simulink model "h3p1_sim"  (R2022b)
settings: Solver=VariableStepAuto  StartTime=0.0  StopTime=Tf  RelTol=1e-3
undefined symbols (not defined in the file): J, Jw, kd_pitch, kd_roll, kd_yaw, kp_pitch, kp_roll, kp_yaw, mu, q_inertial2body_0, q_inertial2body_f, r_inertial_0, v_inertial_0, w_b_0, w_b_nom, X_rw_in_body
libraries: matrix_library x1
settings Model: Creator=corey  LastModifiedBy=corey
settings DebuggingCC: UnconnectedInputMsg=warning  UnconnectedOutputMsg=warning  UnconnectedLineMsg=warning
settings ModelReferenceCC: EnableRefExpFcnMdlSchedulingChecks=on
settings RTWCC: DLArmComputeVersion=19.05

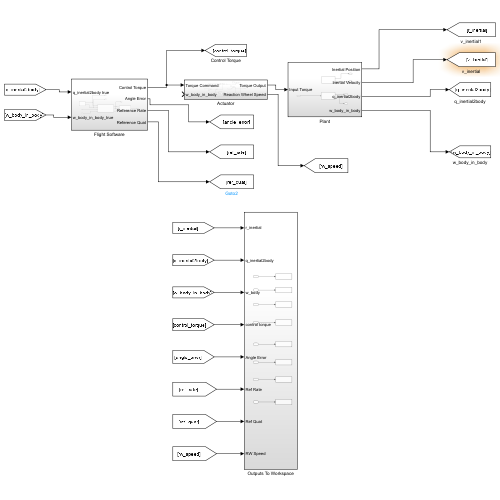
[thumbnail: Simulink's stored preview of the top-level diagram]
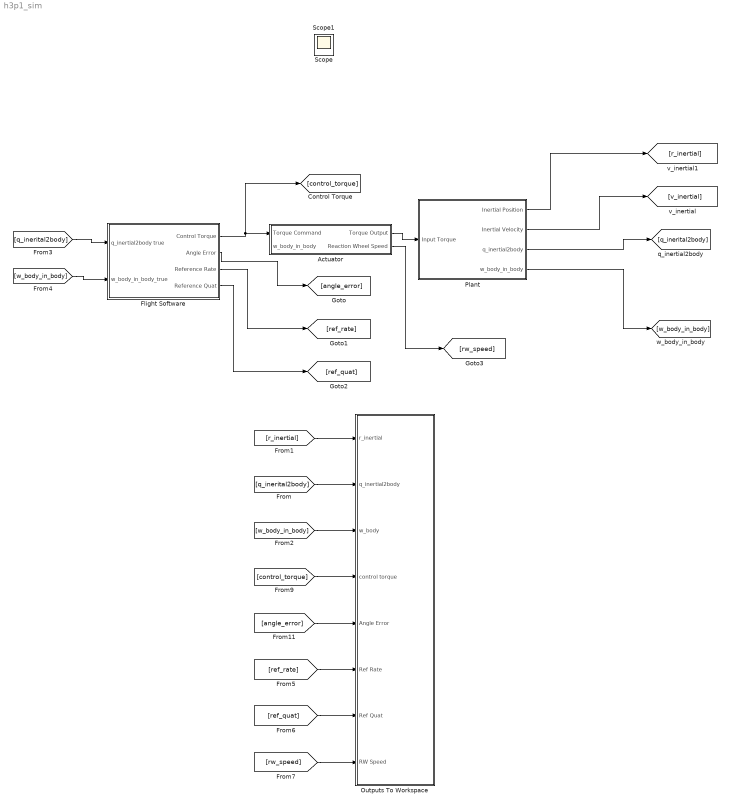
== system h3p1_sim ==
  Actuator : Subsystem
  Flight Software : Subsystem
  Outputs To Workspace : Subsystem
  Plant : Subsystem
  Scope : Scope
  Scope1 : Scope
  wires:
  Plant/4(w_body_in_body) -> [w_body_in_body]
  Plant/3(q_inertial2body) -> [q_inerital2body]
  Plant/2(Inertial Velocity) -> [v_inertial]
  Plant/1(Inertial Position) -> [r_inertial]
  [q_inerital2body] -> Outputs To Workspace/2(q_inertial2body)
  [w_body_in_body] -> Outputs To Workspace/3(w_body)
  [r_inertial] -> Outputs To Workspace/1(r_inertial)
  [control_torque] -> Outputs To Workspace/4(control torque)
  Flight Software/1(Control Torque) -> Actuator/1(Torque Command), [control_torque]
  [angle_error] -> Outputs To Workspace/5(Angle Error)
  Actuator/1(Torque Output) -> Plant/1(Input Torque)
  Flight Software/2(Angle Error) -> [angle_error]
  [q_inerital2body] -> Flight Software/1(q_inertial2body true)
  [w_body_in_body] -> Flight Software/2(w_body_in_body_true)
  Flight Software/3(Reference Rate) -> [ref_rate]
  Flight Software/4(Reference Quat) -> [ref_quat]
  [ref_rate] -> Outputs To Workspace/6(Ref Rate)
  [ref_quat] -> Outputs To Workspace/7(Ref Quat)
  Actuator/2(Reaction Wheel Speed) -> [rw_speed]
  [rw_speed] -> Outputs To Workspace/8(RW Speed)

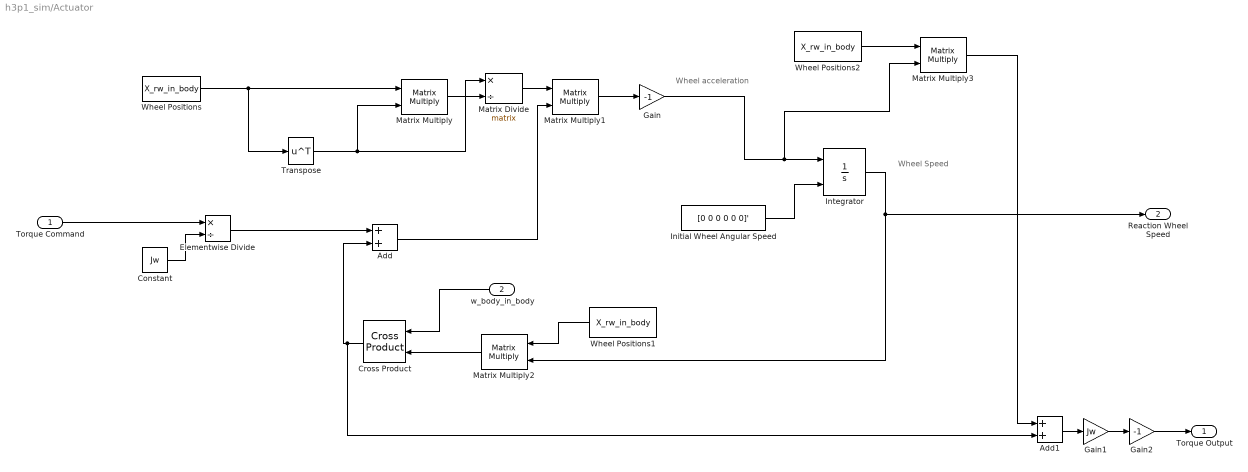
== system h3p1_sim/Actuator ==
  note: Wheel Speed
  note: Wheel acceleration
  Torque Command : Inport
  w_body_in_body : Inport  Port=2
  Add : Sum
  Add1 : Sum
  Constant : Constant  Value=Jw
  Cross Product : matrix_library/Cross Product
  Elementwise Divide : Product  Inputs=*/
  Gain : Gain  Gain=-1
  Gain1 : Gain  Gain=Jw
  Gain2 : Gain  Gain=-1
  Initial Wheel Angular Speed : Constant  Value=[0 0 0 0 0 0]'
  Integrator : Integrator  InitialConditionSource=external
  Matrix Divide : Product  Inputs=*/  Multiplication=Matrix(*)
  Matrix Multiply{,1..3} (4 alike) : Product  Multiplication=Matrix(*)
  Transpose : Math  Operator=transpose
  Wheel Positions : Constant  Value=X_rw_in_body
  Wheel Positions1 : Constant  Value=X_rw_in_body
  Wheel Positions2 : Constant  Value=X_rw_in_body
  Torque Output : Outport
  Reaction Wheel Speed : Outport  Port=2
  wires:
  Initial Wheel Angular Speed/1 -> Integrator/2
  Wheel Positions/1 -> Matrix Multiply/1, Transpose/1
  Transpose/1 -> Matrix Divide/1, Matrix Multiply/2
  Matrix Multiply/1 -> Matrix Divide/2
  Matrix Divide/1 -> Matrix Multiply1/1
  Torque Command/1 -> Elementwise Divide/1
  Constant/1 -> Elementwise Divide/2
  Elementwise Divide/1 -> Add/1
  Integrator/1 -> Reaction Wheel Speed/1, Matrix Multiply2/2
  Wheel Positions1/1 -> Matrix Multiply2/1
  w_body_in_body/1 -> Cross Product/1
  Matrix Multiply2/1 -> Cross Product/2
  Add/1 -> Matrix Multiply1/2
  Matrix Multiply1/1 -> Gain/1
  Gain/1 -> Matrix Multiply3/2, Integrator/1
  Cross Product/1 -> Add1/2, Add/2
  Add1/1 -> Gain1/1
  Wheel Positions2/1 -> Matrix Multiply3/1
  Matrix Multiply3/1 -> Add1/1
  Gain1/1 -> Gain2/1
  Gain2/1 -> Torque Output/1

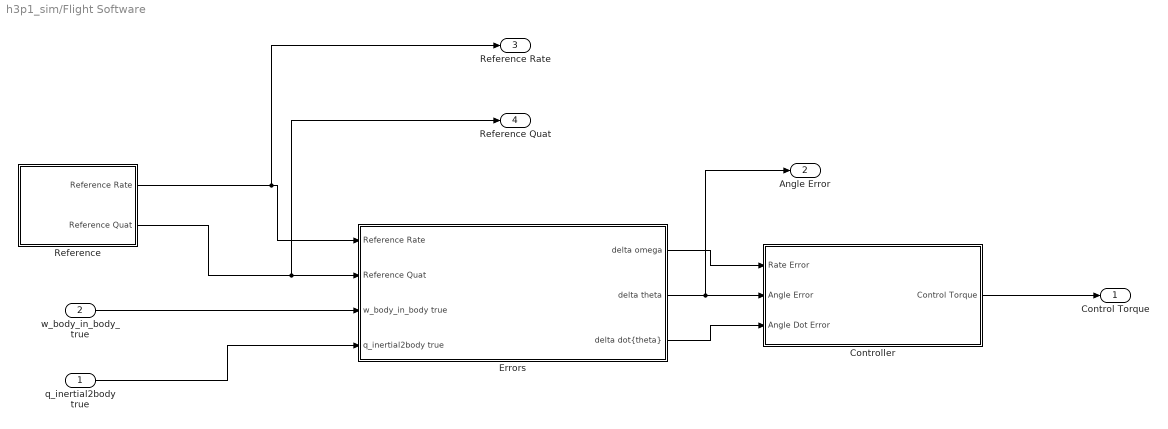
== system h3p1_sim/Flight Software ==
  q_inertial2body true : Inport
  w_body_in_body_true : Inport  Port=2
  Controller : Subsystem
  Errors : Subsystem
  Reference : Subsystem
  Control Torque : Outport
  Angle Error : Outport  Port=2
  Reference Rate : Outport  Port=3
  Reference Quat : Outport  Port=4
  wires:
  Controller/1(Control Torque) -> Control Torque/1
  Errors/1(delta omega) -> Controller/1(Rate Error)
  Errors/2(delta theta) -> Angle Error/1, Controller/2(Angle Error)
  Errors/3("delta dot{theta}") -> Controller/3(Angle Dot Error)
  q_inertial2body true/1 -> Errors/4(q_inertial2body true)
  w_body_in_body_true/1 -> Errors/3(w_body_in_body true)
  Reference/1(Reference Rate) -> Reference Rate/1, Errors/1(Reference Rate)
  Reference/2(Reference Quat) -> Reference Quat/1, Errors/2(Reference Quat)

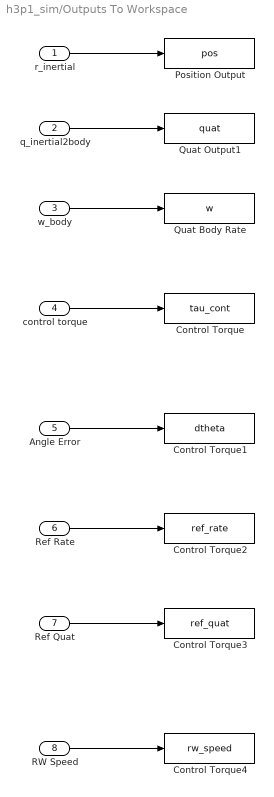
== system h3p1_sim/Outputs To Workspace ==
  r_inertial : Inport
  q_inertial2body : Inport  Port=2
  w_body : Inport  Port=3
  control torque : Inport  Port=4
  Angle Error : Inport  Port=5
  Ref Rate : Inport  Port=6
  Ref Quat : Inport  Port=7
  RW Speed : Inport  Port=8
  Control Torque : ToWorkspace  VariableName=tau_cont  SampleTime=-1
  Control Torque1 : ToWorkspace  VariableName=dtheta  SampleTime=-1
  Control Torque2 : ToWorkspace  VariableName=ref_rate  SampleTime=-1
  Control Torque3 : ToWorkspace  VariableName=ref_quat  SampleTime=-1
  Control Torque4 : ToWorkspace  VariableName=rw_speed  SampleTime=-1
  Position Output : ToWorkspace  VariableName=pos  SampleTime=-1
  Quat Body Rate : ToWorkspace  VariableName=w  SampleTime=-1
  Quat Output1 : ToWorkspace  VariableName=quat  SampleTime=-1
  wires:
  r_inertial/1 -> Position Output/1
  w_body/1 -> Quat Body Rate/1
  q_inertial2body/1 -> Quat Output1/1
  control torque/1 -> Control Torque/1
  Angle Error/1 -> Control Torque1/1
  Ref Rate/1 -> Control Torque2/1
  Ref Quat/1 -> Control Torque3/1
  RW Speed/1 -> Control Torque4/1

== system h3p1_sim/Plant ==
  Input Torque : Inport
  Attitude Dynamics : Subsystem
  Position Dynamics : Subsystem
  Inertial Position : Outport
  Inertial Velocity : Outport  Port=2
  q_inertial2body : Outport  Port=3
  w_body_in_body : Outport  Port=4
  wires:
  Input Torque/1 -> Attitude Dynamics/1(Input Torque)
  Position Dynamics/1(Inertial Position) -> Inertial Position/1
  Position Dynamics/2(Inertial Velocity) -> Inertial Velocity/1
  Attitude Dynamics/1(q_inertial2body) -> q_inertial2body/1
  Attitude Dynamics/2(w_body_in_body) -> w_body_in_body/1

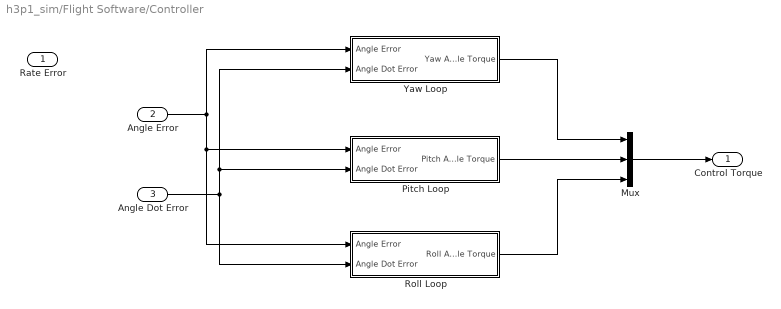
== system h3p1_sim/Flight Software/Controller ==
  Rate Error : Inport
  Angle Error : Inport  Port=2
  Angle Dot Error : Inport  Port=3
  Mux : Mux  Inputs=3
  Pitch Loop : Subsystem
  Roll Loop : Subsystem
  Yaw Loop : Subsystem
  Control Torque : Outport
  wires:
  Angle Error/1 -> Pitch Loop/1(Angle Error), Roll Loop/1(Angle Error), Yaw Loop/1(Angle Error)
  Angle Dot Error/1 -> Pitch Loop/2(Angle Dot Error), Yaw Loop/2(Angle Dot Error), Roll Loop/2(Angle Dot Error)
  Mux/1 -> Control Torque/1
  Yaw Loop/1(Yaw Angle Torque) -> Mux/1
  Pitch Loop/1(Pitch Angle Torque) -> Mux/2
  Roll Loop/1(Roll Angle Torque) -> Mux/3

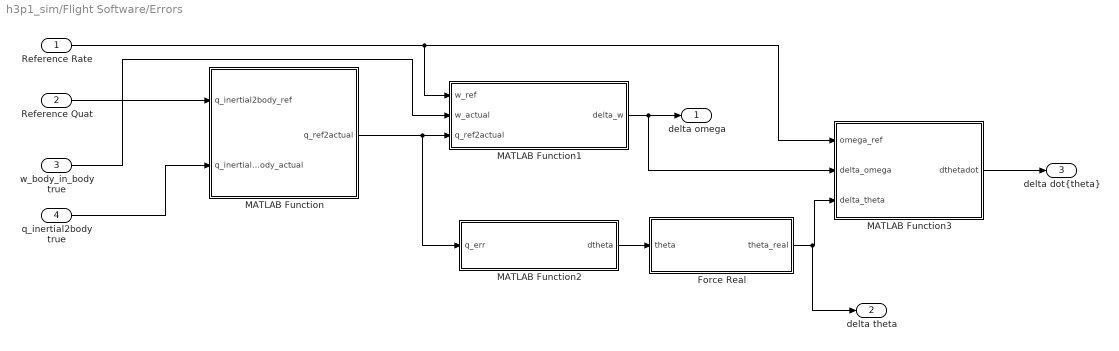
== system h3p1_sim/Flight Software/Errors ==
  Reference Rate : Inport
  Reference Quat : Inport  Port=2
  w_body_in_body true : Inport  Port=3
  q_inertial2body true : Inport  Port=4
  Force Real : MATLAB Function  TreatAsAtomicUnit=on
  MATLAB Function : MATLAB Function  TreatAsAtomicUnit=on
  MATLAB Function1 : MATLAB Function  TreatAsAtomicUnit=on
  MATLAB Function2 : MATLAB Function  TreatAsAtomicUnit=on
  MATLAB Function3 : MATLAB Function  TreatAsAtomicUnit=on
  delta omega : Outport
  delta theta : Outport  Port=2
  "delta dot{theta}" : Outport  Port=3
  wires:
  Reference Quat/1 -> MATLAB Function/1(q_inertial2body_ref)
  q_inertial2body true/1 -> MATLAB Function/2(q_inertial2body_actual)
  MATLAB Function/1(q_ref2actual) -> MATLAB Function2/1(q_err), MATLAB Function1/3(q_ref2actual)
  Reference Rate/1 -> MATLAB Function3/1(omega_ref), MATLAB Function1/1(w_ref)
  w_body_in_body true/1 -> MATLAB Function1/2(w_actual)
  MATLAB Function1/1(delta_w) -> MATLAB Function3/2(delta_omega), delta omega/1
  MATLAB Function3/1(dthetadot) -> "delta dot{theta}"/1
  MATLAB Function2/1(dtheta) -> Force Real/1(theta)
  Force Real/1(theta_real) -> delta theta/1, MATLAB Function3/3(delta_theta)

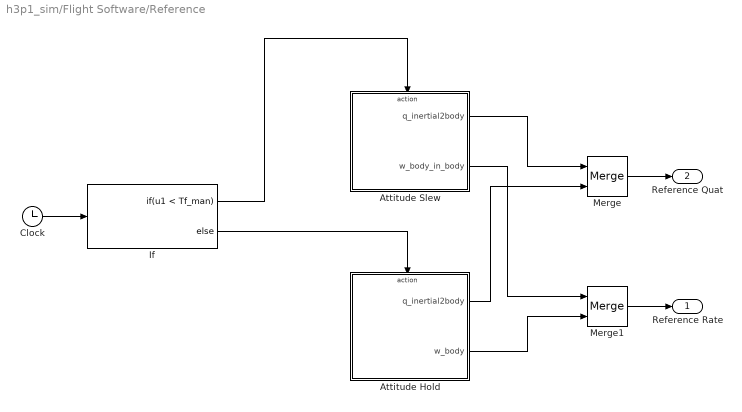
== system h3p1_sim/Flight Software/Reference ==
  Attitude Hold : Subsystem  TreatAsAtomicUnit=on
  Attitude Slew : Subsystem  TreatAsAtomicUnit=on
  Clock : Clock
  If : If  IfExpression=u1 < Tf_man
  Merge : Merge
  Merge1 : Merge
  Reference Rate : Outport
  Reference Quat : Outport  Port=2
  wires:
  Clock/1 -> If/1
  If/1 -> Attitude Slew/Action
  If/2 -> Attitude Hold/Action
  Attitude Slew/1(q_inertial2body) -> Merge/1
  Attitude Hold/1(q_inertial2body) -> Merge/2
  Merge/1 -> Reference Quat/1
  Merge1/1 -> Reference Rate/1
  Attitude Slew/2(w_body_in_body) -> Merge1/1
  Attitude Hold/2(w_body) -> Merge1/2

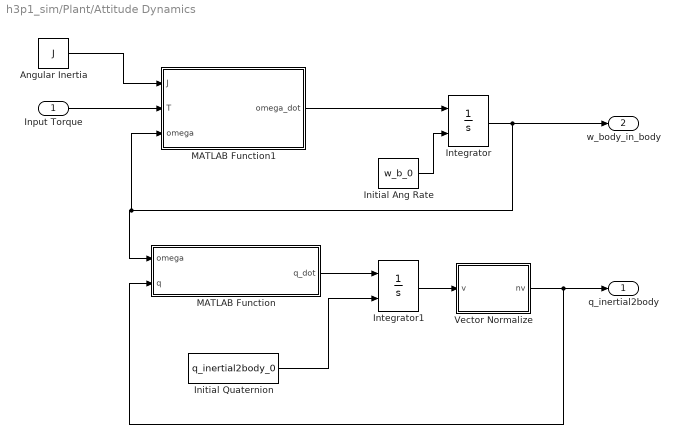
== system h3p1_sim/Plant/Attitude Dynamics ==
  Input Torque : Inport
  Angular Inertia : Constant  Value=J
  Initial Ang Rate : Constant  Value=w_b_0
  Initial Quaternion : Constant  Value=q_inertial2body_0
  Integrator : Integrator  InitialConditionSource=external
  Integrator1 : Integrator  InitialConditionSource=external
  MATLAB Function : MATLAB Function  TreatAsAtomicUnit=on
  MATLAB Function1 : MATLAB Function  TreatAsAtomicUnit=on
  Vector Normalize : MATLAB Function  TreatAsAtomicUnit=on
  q_inertial2body : Outport
  w_body_in_body : Outport  Port=2
  wires:
  Integrator/1 -> MATLAB Function1/3(omega), MATLAB Function/1(omega), w_body_in_body/1
  MATLAB Function1/1(omega_dot) -> Integrator/1
  Initial Ang Rate/1 -> Integrator/2
  MATLAB Function/1(q_dot) -> Integrator1/1
  Initial Quaternion/1 -> Integrator1/2
  Integrator1/1 -> Vector Normalize/1(v)
  Vector Normalize/1(nv) -> MATLAB Function/2(q), q_inertial2body/1
  Input Torque/1 -> MATLAB Function1/2(T)
  Angular Inertia/1 -> MATLAB Function1/1(J)

== system h3p1_sim/Plant/Position Dynamics ==
  Gravity Constant : Constant  Value=mu
  Initial Position : Constant  Value=r_inertial_0
  Initial Velocity : Constant  Value=v_inertial_0
  Integrator : Integrator  InitialConditionSource=external  InitialCondition=[6871, 0, 0]'
  Integrator1 : Integrator  InitialConditionSource=external  InitialCondition=[0, 7.6166, 0]'
  Vector Norm : MATLAB Function  TreatAsAtomicUnit=on
  Inertial Position : Outport
  Inertial Velocity : Outport  Port=2
  wires:
  Integrator/1 -> Vector Norm/1(r), Inertial Position/1  "Position"
  Integrator1/1 -> Inertial Velocity/1, Integrator/1  "Velocity"
  Vector Norm/1(a) -> Integrator1/1  "Accel"
  Gravity Constant/1 -> Vector Norm/2(mu)
  Initial Velocity/1 -> Integrator1/2
  Initial Position/1 -> Integrator/2

== system h3p1_sim/Flight Software/Controller/Pitch Loop ==
  Angle Error : Inport
  Angle Dot Error : Inport  Port=2
  PD Controller : Subsystem
  Pitch Angle Torque : Outport
  wires:
  Angle Error/1 -> PD Controller/1(Angle Error)
  Angle Dot Error/1 -> PD Controller/2(Angle Error Dot)
  PD Controller/1(Pitch Angle Torque) -> Pitch Angle Torque/1

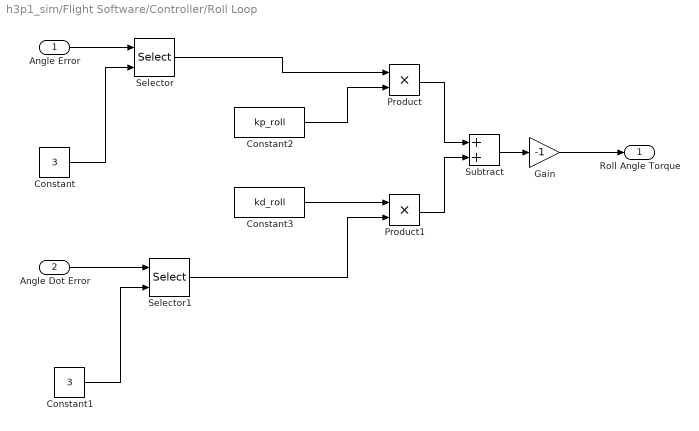
== system h3p1_sim/Flight Software/Controller/Roll Loop ==
  Angle Error : Inport
  Angle Dot Error : Inport  Port=2
  Constant : Constant  Value=3
  Constant1 : Constant  Value=3
  Constant2 : Constant  Value=kp_roll
  Constant3 : Constant  Value=kd_roll
  Gain : Gain  Gain=-1
  Product : Product
  Product1 : Product
  Selector : Selector  InputPortWidth=3  IndexOptions=Index vector (port)  Indices=[1 3]  OutputSizes=1
  Selector1 : Selector  InputPortWidth=3  IndexOptions=Index vector (port)  Indices=[1 3]  OutputSizes=1
  Subtract : Sum
  Roll Angle Torque : Outport
  wires:
  Angle Error/1 -> Selector/1
  Constant/1 -> Selector/2
  Constant1/1 -> Selector1/2
  Angle Dot Error/1 -> Selector1/1
  Selector/1 -> Product/1
  Constant2/1 -> Product/2
  Constant3/1 -> Product1/1
  Selector1/1 -> Product1/2
  Product/1 -> Subtract/1
  Product1/1 -> Subtract/2
  Subtract/1 -> Gain/1
  Gain/1 -> Roll Angle Torque/1

== system h3p1_sim/Flight Software/Controller/Yaw Loop ==
  Angle Error : Inport
  Angle Dot Error : Inport  Port=2
  PD Controller : Subsystem
  Yaw Angle Torque : Outport
  wires:
  Angle Error/1 -> PD Controller/1(Angle Error)
  Angle Dot Error/1 -> PD Controller/2(Angle Error Dot)
  PD Controller/1(Yaw Angle Torque) -> Yaw Angle Torque/1

== system h3p1_sim/Flight Software/Reference/Attitude Hold ==
  Action Port : ActionPort  ActionPortLabel=else
  Constant : Constant  Value=q_inertial2body_f
  Constant1 : Constant  Value=[0 0 0]'
  q_inertial2body : Outport
  w_body : Outport  Port=2
  wires:
  Constant/1 -> q_inertial2body/1
  Constant1/1 -> w_body/1

== system h3p1_sim/Flight Software/Reference/Attitude Slew ==
  Action Port : ActionPort  ActionPortLabel=if(u1 < Tf_man)
  Constant : Constant  Value=[0 0 0]'
  Reference Plant : Subsystem
  q_inertial2body : Outport
  w_body_in_body : Outport  Port=2
  wires:
  Constant/1 -> Reference Plant/1(Input Torque)
  Reference Plant/3(q_inertial2body) -> q_inertial2body/1
  Reference Plant/4(w_body_in_body) -> w_body_in_body/1

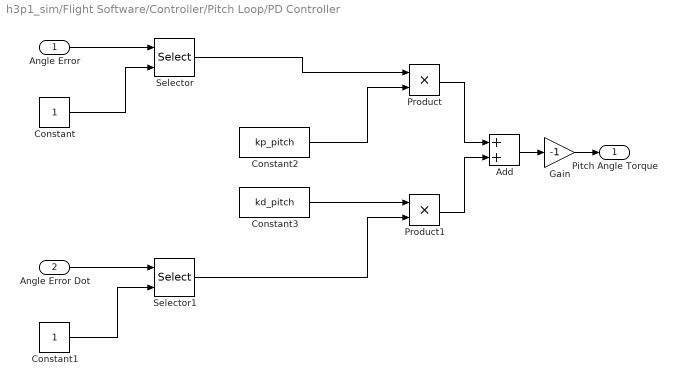
== system h3p1_sim/Flight Software/Controller/Pitch Loop/PD Controller ==
  Angle Error : Inport
  Angle Error Dot : Inport  Port=2
  Add : Sum
  Constant : Constant
  Constant1 : Constant
  Constant2 : Constant  Value=kp_pitch
  Constant3 : Constant  Value=kd_pitch
  Gain : Gain  Gain=-1
  Product : Product
  Product1 : Product
  Selector : Selector  InputPortWidth=3  IndexOptions=Index vector (port)  Indices=[1 3]  OutputSizes=1
  Selector1 : Selector  InputPortWidth=3  IndexOptions=Index vector (port)  Indices=[1 3]  OutputSizes=1
  Pitch Angle Torque : Outport
  wires:
  Constant2/1 -> Product/2
  Constant3/1 -> Product1/1
  Selector1/1 -> Product1/2
  Constant1/1 -> Selector1/2
  Angle Error Dot/1 -> Selector1/1
  Constant/1 -> Selector/2
  Product/1 -> Add/1
  Selector/1 -> Product/1
  Product1/1 -> Add/2
  Angle Error/1 -> Selector/1
  Add/1 -> Gain/1
  Gain/1 -> Pitch Angle Torque/1

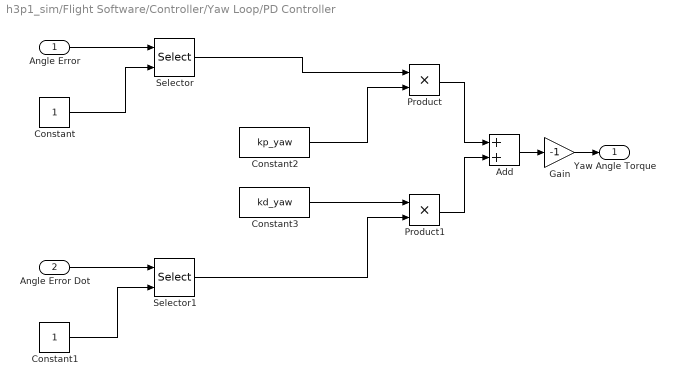
== system h3p1_sim/Flight Software/Controller/Yaw Loop/PD Controller ==
  Angle Error : Inport
  Angle Error Dot : Inport  Port=2
  Add : Sum
  Constant : Constant
  Constant1 : Constant
  Constant2 : Constant  Value=kp_yaw
  Constant3 : Constant  Value=kd_yaw
  Gain : Gain  Gain=-1
  Product : Product
  Product1 : Product
  Selector : Selector  InputPortWidth=3  IndexOptions=Index vector (port)  Indices=[1 3]  OutputSizes=1
  Selector1 : Selector  InputPortWidth=3  IndexOptions=Index vector (port)  Indices=[1 3]  OutputSizes=1
  Yaw Angle Torque : Outport
  wires:
  Constant2/1 -> Product/2
  Constant3/1 -> Product1/1
  Selector1/1 -> Product1/2
  Constant1/1 -> Selector1/2
  Angle Error Dot/1 -> Selector1/1
  Constant/1 -> Selector/2
  Product/1 -> Add/1
  Selector/1 -> Product/1
  Product1/1 -> Add/2
  Angle Error/1 -> Selector/1
  Add/1 -> Gain/1
  Gain/1 -> Yaw Angle Torque/1

== system h3p1_sim/Flight Software/Reference/Attitude Slew/Reference Plant ==
  Input Torque : Inport
  Attitude Dynamics : Subsystem
  Position Dynamics : Subsystem
  Inertial Position : Outport
  Inertial Velocity : Outport  Port=2
  q_inertial2body : Outport  Port=3
  w_body_in_body : Outport  Port=4
  wires:
  Input Torque/1 -> Attitude Dynamics/1(Input Torque)
  Position Dynamics/1(Inertial Position) -> Inertial Position/1
  Position Dynamics/2(Inertial Velocity) -> Inertial Velocity/1
  Attitude Dynamics/1(q_inertial2body) -> q_inertial2body/1
  Attitude Dynamics/2(w_body_in_body) -> w_body_in_body/1

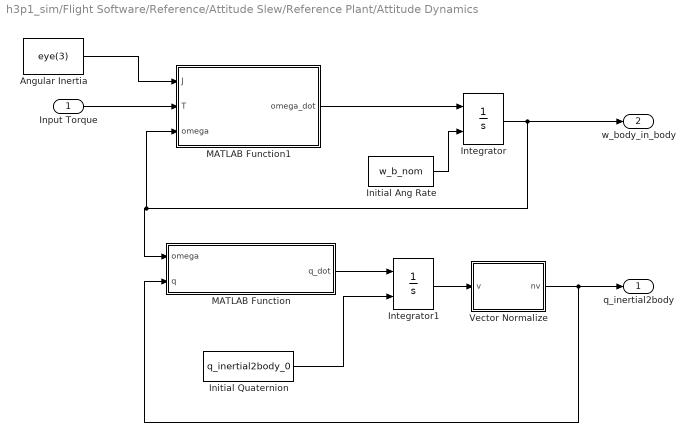
== system h3p1_sim/Flight Software/Reference/Attitude Slew/Reference Plant/Attitude Dynamics ==
  Input Torque : Inport
  Angular Inertia : Constant  Value=eye(3)
  Initial Ang Rate : Constant  Value=w_b_nom
  Initial Quaternion : Constant  Value=q_inertial2body_0
  Integrator : Integrator  InitialConditionSource=external
  Integrator1 : Integrator  InitialConditionSource=external
  MATLAB Function : MATLAB Function  TreatAsAtomicUnit=on
  MATLAB Function1 : MATLAB Function  TreatAsAtomicUnit=on
  Vector Normalize : MATLAB Function  TreatAsAtomicUnit=on
  q_inertial2body : Outport
  w_body_in_body : Outport  Port=2
  wires:
  Integrator/1 -> MATLAB Function1/3(omega), MATLAB Function/1(omega), w_body_in_body/1
  MATLAB Function1/1(omega_dot) -> Integrator/1
  Initial Ang Rate/1 -> Integrator/2
  MATLAB Function/1(q_dot) -> Integrator1/1
  Initial Quaternion/1 -> Integrator1/2
  Integrator1/1 -> Vector Normalize/1(v)
  Vector Normalize/1(nv) -> MATLAB Function/2(q), q_inertial2body/1
  Input Torque/1 -> MATLAB Function1/2(T)
  Angular Inertia/1 -> MATLAB Function1/1(J)

== system h3p1_sim/Flight Software/Reference/Attitude Slew/Reference Plant/Position Dynamics ==
  Gravity Constant : Constant  Value=mu
  Initial Position : Constant  Value=r_inertial_0
  Initial Velocity : Constant  Value=v_inertial_0
  Integrator : Integrator  InitialConditionSource=external  InitialCondition=[6871, 0, 0]'
  Integrator1 : Integrator  InitialConditionSource=external  InitialCondition=[0, 7.6166, 0]'
  Vector Norm : MATLAB Function  TreatAsAtomicUnit=on
  Inertial Position : Outport
  Inertial Velocity : Outport  Port=2
  wires:
  Integrator/1 -> Vector Norm/1(r), Inertial Position/1  "Position"
  Integrator1/1 -> Inertial Velocity/1, Integrator/1  "Velocity"
  Vector Norm/1(a) -> Integrator1/1  "Accel"
  Gravity Constant/1 -> Vector Norm/2(mu)
  Initial Velocity/1 -> Integrator1/2
  Initial Position/1 -> Integrator/2

== matlab function h3p1_sim/Flight Software/Errors/Force Real ==
  data: theta input; theta_real output
function theta_real = ForceReal(theta)

theta_real = real(theta);

== matlab function h3p1_sim/Plant/Position Dynamics/Vector Norm ==
  data: r input; a output; mu input
function a = TwoBodyGrav(r,mu)

nr = norm(r);
a = -mu*r/(nr^3);

== matlab function h3p1_sim/Plant/Attitude Dynamics/MATLAB Function1 ==
  data: J input; omega_dot output; T input; omega input
function omega_dot = OmegaEvolution(J, T, omega)
omega_dot = J\(T - cross(omega, J*omega));

== matlab function h3p1_sim/Plant/Attitude Dynamics/Vector Normalize ==
  data: v input; nv output
function nv = NormVec(v)

nv = v/norm(v);

== matlab function h3p1_sim/Flight Software/Reference/Attitude Slew/Reference Plant/Attitude Dynamics/MATLAB Function ==
  data: omega input; q_dot output; q input
function q_dot = QuaternionEvolution(omega, q)
intermed = [omega; 0];
q_dot = 0.5*QuatProduct(intermed,q);

== matlab function h3p1_sim/Flight Software/Reference/Attitude Slew/Reference Plant/Attitude Dynamics/MATLAB Function1 ==
  data: J input; omega_dot output; T input; omega input
function omega_dot = OmegaEvolution(J, T, omega)
omega_dot = J\(T - cross(omega, J*omega));

== matlab function h3p1_sim/Flight Software/Reference/Attitude Slew/Reference Plant/Attitude Dynamics/Vector Normalize ==
  data: v input; nv output
function nv = NormVec(v)

nv = v/norm(v);

== matlab function h3p1_sim/Flight Software/Errors/MATLAB Function ==
  data: q_inertial2body_ref input; q_ref2actual output; q_inertial2body_actual input
function q_ref2actual = ErrorQuat(q_inertial2body_ref, q_inertial2body_actual)

q_ref2actual = QuatProduct(q_inertial2body_actual,QuatInv(q_inertial2body_ref));

% Force normalization
q_ref2actual = q_ref2actual/norm(q_ref2actual);

== matlab function h3p1_sim/Flight Software/Errors/MATLAB Function1 ==
  data: w_ref input; delta_w output; w_actual input; q_ref2actual input
function delta_w = ErrorRate(w_ref, w_actual, q_ref2actual)

delta_w = w_actual - QuatTransform(q_ref2actual,w_ref);

== matlab function h3p1_sim/Flight Software/Errors/MATLAB Function2 ==
  data: q_err input; dtheta output
function dtheta = ErrorQuat2ErrorAngle(q_err)

% Quaternion components
q_v = real(q_err(1:3));
q_s = real(q_err(4));

dtheta = [atan2(q_v(1),q_s);
    atan2(q_v(2),q_s);
    atan2(q_v(3),q_s)];

== matlab function h3p1_sim/Flight Software/Errors/MATLAB Function3 ==
  data: omega_ref input; dthetadot output; delta_omega input; delta_theta input
function dthetadot = ErrorThetaDot(omega_ref, delta_omega, delta_theta)

dthetadot = delta_omega - cross(omega_ref,delta_theta);

== matlab function h3p1_sim/Plant/Attitude Dynamics/MATLAB Function ==
  data: omega input; q_dot output; q input
function q_dot = QuaternionEvolution(omega, q)
intermed = [omega; 0];
q_dot = 0.5*QuatProduct(intermed,q);

== matlab function h3p1_sim/Flight Software/Reference/Attitude Slew/Reference Plant/Position Dynamics/Vector Norm ==
  data: r input; a output; mu input
function a = TwoBodyGrav(r,mu)

nr = norm(r);
a = -mu*r/(nr^3);
